simulink model "sim_adaptive_rbf_nonlinear_system"  (R2023a)
settings: Solver=VariableStepAuto  StartTime=0.0  StopTime=30  RelTol=1e-3
settings Model: Creator=ACCENT  LastModifiedBy=ACCENT

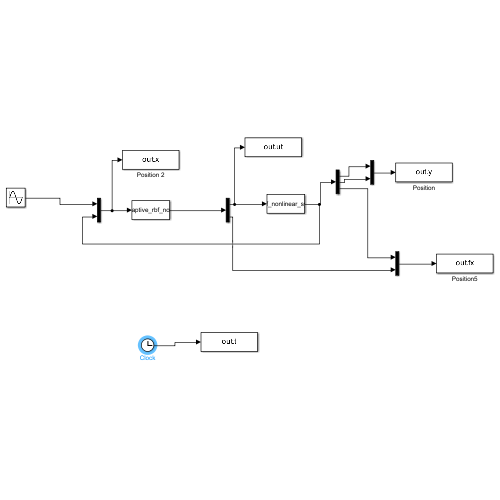
[thumbnail: Simulink's stored preview of the top-level diagram]
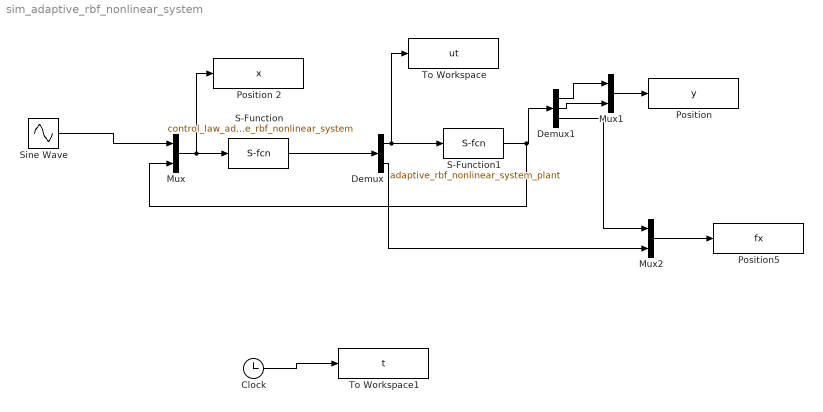
== system sim_adaptive_rbf_nonlinear_system ==
  Clock : Clock
      settings: Decimation=30
  Demux : Demux  Outputs=2
  Demux1 : Demux  Outputs=3
  Mux : Mux  Inputs=2
  Mux1 : Mux  Inputs=2
  Mux2 : Mux  Inputs=2
  Position : ToWorkspace  VariableName=y  SampleTime=-1
  Position 2 : ToWorkspace  VariableName=x  SampleTime=-1
  Position5 : ToWorkspace  VariableName=fx  SampleTime=-1
  S-Function : S-Function  FunctionName=control_law_adaptive_rbf_nonlinear_system  SFunctionDeploymentMode=off  EnableBusSupport=off
  S-Function1 : S-Function  FunctionName=adaptive_rbf_nonlinear_system_plant  SFunctionDeploymentMode=off  EnableBusSupport=off
  Sine Wave : Sin  Amplitude=0.1  SampleTime=0
  To Workspace : ToWorkspace  VariableName=ut  SampleTime=-1
  To Workspace1 : ToWorkspace  VariableName=t  SampleTime=-1
  wires:
  Mux2/1 -> Position5/1
  Clock/1 -> To Workspace1/1
  Sine Wave/1 -> Mux/1
  Mux/1 -> Position 2/1, S-Function/1
  S-Function/1 -> Demux/1
  Demux/1 -> S-Function1/1, To Workspace/1
  Demux/2 -> Mux2/2
  S-Function1/1 -> Mux/2, Demux1/1
  Demux1/1 -> Mux1/1
  Demux1/2 -> Mux1/2
  Demux1/3 -> Mux2/1
  Mux1/1 -> Position/1
